simulink model "APER1"  (R2017a)
settings: Solver=VariableStepAuto  StartTime=0.0  StopTime=10  MaxStep=0.001000001  MinStep=0.001  RelTol=1e-5
undefined symbols (not defined in the file): k, T, w
settings Model: Creator=User  LastModifiedBy=User

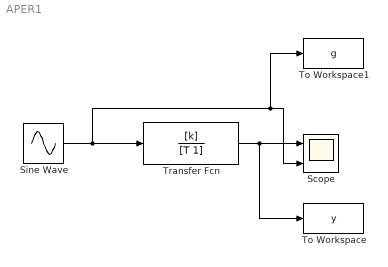
== system APER1 ==
  Scope : Scope  NumInputPorts=2
  Sine Wave : Sin  Frequency=w  SampleTime=0
  To Workspace : ToWorkspace  VariableName=y  SampleTime=-1
  To Workspace1 : ToWorkspace  VariableName=g  SampleTime=-1
  Transfer Fcn : TransferFcn  Numerator=[k]  Denominator=[T 1]
  wires:
  Sine Wave/1 -> To Workspace1/1, Scope/2, Transfer Fcn/1
  Transfer Fcn/1 -> To Workspace/1, Scope/1
